simulink model "model_simulink"  (R2019b)
settings: Solver=VariableStepAuto  StartTime=0.0  StopTime=5  RelTol=1e-3
settings Model: Creator=Alexander  LastModifiedBy=Alexander

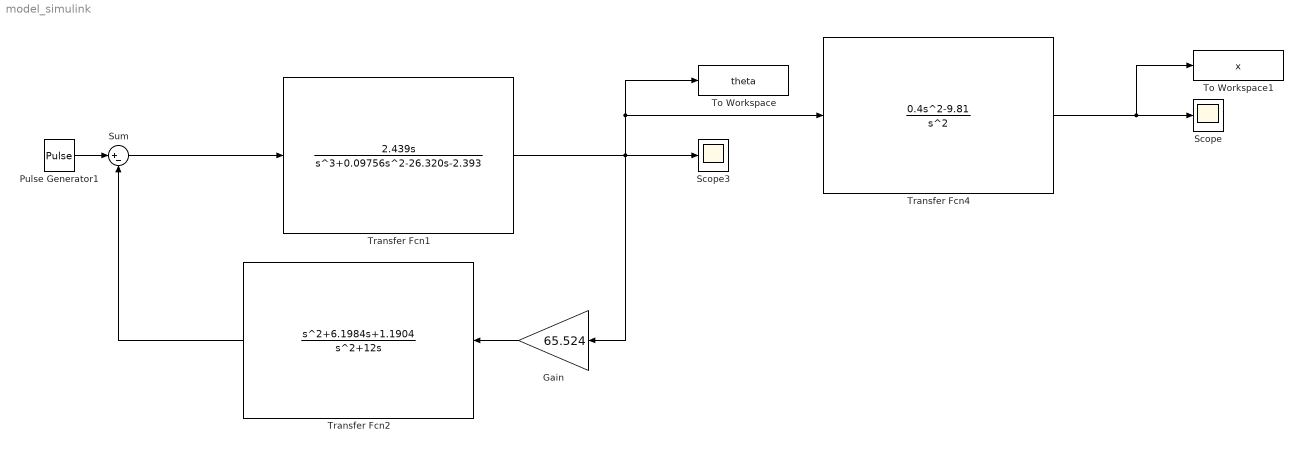
== system model_simulink ==
  Gain : Gain  Gain=65.524
  Pulse Generator1 : DiscretePulseGenerator  PulseType=Time based  Amplitude=10000  Period=1000  PulseWidth=0.00001
  Scope : Scope
  Scope3 : Scope
  Sum : Sum  Inputs=|+-
  To Workspace : ToWorkspace  VariableName=theta  SaveFormat=Structure With Time  SampleTime=-1
  To Workspace1 : ToWorkspace  VariableName=x  SaveFormat=Structure With Time  SampleTime=-1
  Transfer Fcn1 : TransferFcn  Numerator=[2.439 0]  Denominator=[1 0.09756 -26.320 -2.393]
  Transfer Fcn2 : TransferFcn  Numerator=[1 6.1984 1.1904]  Denominator=[1 12 0]
  Transfer Fcn4 : TransferFcn  Numerator=[0.4 0 -9.81]  Denominator=[1 0 0]
  wires:
  Pulse Generator1/1 -> Sum/1
  Transfer Fcn1/1 -> To Workspace/1, Transfer Fcn4/1, Gain/1, Scope3/1
  Sum/1 -> Transfer Fcn1/1
  Gain/1 -> Transfer Fcn2/1
  Transfer Fcn2/1 -> Sum/2
  Transfer Fcn4/1 -> Scope/1, To Workspace1/1
